simulink model "DC_motor_response"  (R2015b)
settings: Solver=VariableStepAuto  StartTime=0.0  StopTime=10.0  FixedStep=0.001  RelTol=1e-3
settings Model: Creator=mgreiff  LastModifiedBy=mgreiff

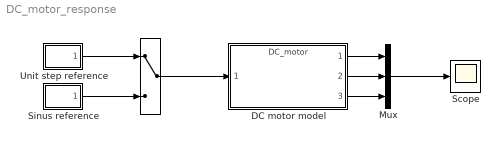
== system DC_motor_response ==
  "   " : ManualSwitch
  DC motor model : ModelReference  ModelNameDialog=DC_motor.slx  SimulationMode=Normal  ModelReferenceVersion=1.7  CopyOfModelName=DC_motor.slx
  Mux : Mux  Inputs=3
  Scope : Scope
  Sinus reference : Subsystem
  Unit step reference : Subsystem
  wires:
  "   "/1 -> DC motor model/1
  DC motor model/1 -> Mux/1
  DC motor model/2 -> Mux/2
  DC motor model/3 -> Mux/3
  Mux/1 -> Scope/1
  Unit step reference/1(voltage) -> "   "/1
  Sinus reference/1(voltage) -> "   "/2

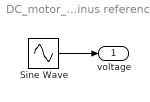
== system DC_motor_response/Sinus reference ==
  Sine Wave : Sin  SampleTime=0
  voltage : Outport
  wires:
  Sine Wave/1 -> voltage/1

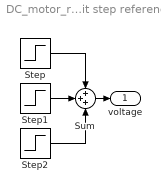
== system DC_motor_response/Unit step reference ==
  Step : Step  Time=0  SampleTime=0
  Step1 : Step  Time=4  After=-2  SampleTime=0
  Step2 : Step  Time=8  SampleTime=0
  Sum : Sum  Inputs=+++
  voltage : Outport
  wires:
  Sum/1 -> voltage/1
  Step1/1 -> Sum/2
  Step2/1 -> Sum/3
  Step/1 -> Sum/1
